simulink model "VehicleSilSimulation"  (R2026a)
settings: configuration reference "standardSILConfigurationParams" (kept outside this file)
StopFcn:
  | fid = fopen('C:\Users\Edison Altamirano\SITLV2\AnelloSummer\optimAeroPX4SIL\HILDiagnostics\logs\session_gtfix1\matlab_error_capture.txt','a'); fprintf(fid, '--- StopFcn fired at %s ---\n', datestr(now)); [m,i] = lasterr(); fprintf(fid, 'lasterr: %s (id: %s)\n', m, i); try; le = lasterror(); fprintf(fid, 'stack:\n'); for k=1:numel(le.stack); fprintf(fid, '  %s line %d\n', le.stack(k).name, le.stack(k).line); end; catch; end; fclose(fid);
values from neighbouring files (symbols this model uses):
  CONTROLLER_RUNTIME = 1    [initVehicleSIL.m]
  stepSize_s = 0.004    [initVehicleSIL.m]
  vehicleParams = evalin('base', 'vehicleParams')    [testVehicleSIL.m]
undefined symbols (not defined in the file or in its folder): actuatorDelay_s, controllerArmed, EngineCommandBus, gpsFreq, heartbeatFreq, opts, Payload, plantSampleTime_s, referenceLatitude_deg, referenceLongitude_deg, SampleTime, ServosCommandBus
libraries: uavmavlinklib x8, simulink x8, instrumentlib x6, flightGearInterfaceLibrary x6, aerolibfltsims x3, sharedtransform x3, px4MAVLinkBridgelib x2, aerolibanimutils x1, hdlsllib x1, dspnetwork x1, robotcorelib x1, uavutilslib x1
(part 2 of 3)

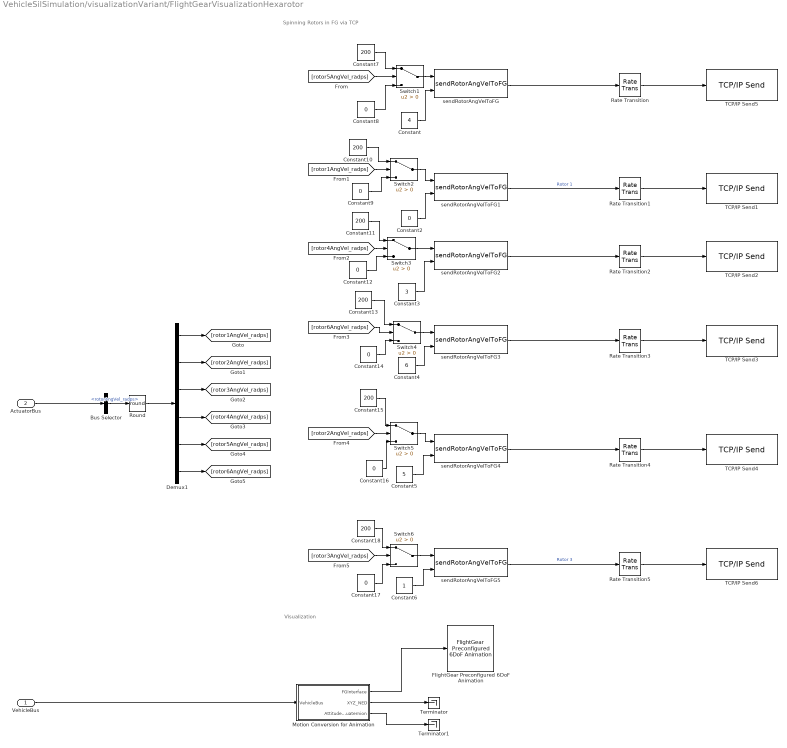
== system VehicleSilSimulation/visualizationVariant/FlightGearVisualizationHexarotor ==
  note: Spinning Rotors in FG via TCP
  note: Visualization
  VehicleBus : Inport
  ActuatorBus : Inport  Port=2  OutDataTypeStr=Bus:ActuatorBus
  Bus Selector : BusSelector  OutputSignals=PropulsionBus.rotorAngVel_radps
  Constant : Constant  Value=4
  Constant{7,10..11,13,15,18} (6 alike) : Constant  Value=200
  Constant{2,8..9,12,14,16..17} (7 alike) : Constant  Value=0
  Constant3 : Constant  Value=3
  Constant4 : Constant  Value=6
  Constant5 : Constant  Value=5
  Constant6 : Constant
  Demux1 : Demux  Outputs=6
  FlightGear Preconfigured 6DoF Animation : aerolibfltsims/FlightGear Preconfigured 6DoF Animation  xFlightGearVersion=v2019.1  DestinationIpAddress=127.0.0.1  DestinationPort=5502  SampleTime=-1  packetVersion=24
  Motion Conversion for Animation : Subsystem
      mask Display:
      | port_label('input',1,'ACBus')
      | port_label('output',1,'\lambda,L,h,\phi,\theta,\psi','texmode','on')
  Rate Transition{,1..5} (6 alike) : RateTransition  OutPortSampleTime=visualizationParams.flightGearFreq_Hz
  Round : Rounding  Operator=round
  Switch{1..6} (6 alike) : Switch  Criteria=u2 > Threshold  SaturateOnIntegerOverflow=off  InputSameDT=off
  TCP/IP Send{1..6} (6 alike) : instrumentlib/TCP//IP Send  Host=127.0.0.1  Port=5400  ByteOrder=big-endian  EnableBlockingMode=off  Timeout=10  TransferDelay=off  SimulateUsing=Interpreted execution
  Terminator : Terminator
  Terminator1 : Terminator
  sendRotorAngVelToFG{,1..5} (6 alike) : flightGearInterfaceLibrary/sendRotorAngVelToFG  SystemSampleTime=-1  VariantActivationTime=update diagram  EmptyChoice=off  PassThrough=off  PassThroughVariantControl=(default)  EmptyChoiceVariantControl=(default)  AllowFlexibleInterface=on  Latency=0  AutoFrameSizeCalculation=off
  wires:
  Motion Conversion for Animation/1(FGInterface) -> FlightGear Preconfigured 6DoF Animation/1
  VehicleBus/1 -> Motion Conversion for Animation/1(VehicleBus)
  Motion Conversion for Animation/2(XYZ_NED) -> Terminator/1
  Motion Conversion for Animation/3(AttitudeQuaternion) -> Terminator1/1
  ActuatorBus/1 -> Bus Selector/1
  Bus Selector/1 -> Round/1  "<rotorAngVel_radps>"
  Demux1/1 -> [rotor1AngVel_radps]
  Demux1/2 -> [rotor2AngVel_radps]
  Demux1/5 -> [rotor5AngVel_radps]
  Demux1/6 -> [rotor6AngVel_radps]
  Demux1/4 -> [rotor4AngVel_radps]
  Demux1/3 -> [rotor3AngVel_radps]
  Constant/1 -> sendRotorAngVelToFG/2
  Constant2/1 -> sendRotorAngVelToFG1/2
  Constant3/1 -> sendRotorAngVelToFG2/2
  Constant4/1 -> sendRotorAngVelToFG3/2
  Constant5/1 -> sendRotorAngVelToFG4/2
  Constant6/1 -> sendRotorAngVelToFG5/2
  Round/1 -> Demux1/1
  sendRotorAngVelToFG4/1 -> Rate Transition4/1
  sendRotorAngVelToFG3/1 -> Rate Transition3/1
  sendRotorAngVelToFG5/1 -> Rate Transition5/1  "Rotor 3"
  sendRotorAngVelToFG1/1 -> Rate Transition1/1  "Rotor 1"
  sendRotorAngVelToFG/1 -> Rate Transition/1
  sendRotorAngVelToFG2/1 -> Rate Transition2/1
  [rotor5AngVel_radps] -> Switch1/2
  Switch1/1 -> sendRotorAngVelToFG/1
  Constant7/1 -> Switch1/1
  Constant8/1 -> Switch1/3
  Switch2/1 -> sendRotorAngVelToFG1/1
  [rotor1AngVel_radps] -> Switch2/2
  Constant9/1 -> Switch2/3
  Constant10/1 -> Switch2/1
  Switch3/1 -> sendRotorAngVelToFG2/1
  [rotor4AngVel_radps] -> Switch3/2
  Constant11/1 -> Switch3/1
  Constant12/1 -> Switch3/3
  Switch4/1 -> sendRotorAngVelToFG3/1
  [rotor6AngVel_radps] -> Switch4/2
  Constant13/1 -> Switch4/1
  Constant14/1 -> Switch4/3
  Switch5/1 -> sendRotorAngVelToFG4/1
  [rotor2AngVel_radps] -> Switch5/2
  Constant15/1 -> Switch5/1
  Constant16/1 -> Switch5/3
  Switch6/1 -> sendRotorAngVelToFG5/1
  [rotor3AngVel_radps] -> Switch6/2
  Constant17/1 -> Switch6/3
  Constant18/1 -> Switch6/1
  Rate Transition/1 -> TCP/IP Send5/1
  Rate Transition1/1 -> TCP/IP Send1/1
  Rate Transition2/1 -> TCP/IP Send2/1
  Rate Transition3/1 -> TCP/IP Send3/1
  Rate Transition4/1 -> TCP/IP Send4/1
  Rate Transition5/1 -> TCP/IP Send6/1

== system VehicleSilSimulation/visualizationVariant/MatlabVisualization ==
  note: Visualization
  VehicleBus : Inport
  Motion Conversion for Animation : Subsystem
      mask Display:
      | port_label('input',1,'ACBus')
      | port_label('output',1,'\lambda,L,h,\phi,\theta,\psi','texmode','on')
  Terminator : Terminator
  UAV Animation : uavutilslib/UAV Animation  NumUAV=1  DynamicUAVConfig=off  UAVType=FixedWing  UAVSize=100  UAVColor=[1 0 0]  UAVTrajectoryAlpha=1  AlwaysShowAnimation=on  AxisLimits=[-Inf Inf;-Inf Inf;-Inf Inf]  TrajectoryBufferSize=100000  InertialZDirection=Down  RotationFormat=Quaternion  DrawMarkers=off  SampleTime=0.04
  wires:
  Motion Conversion for Animation/2(XYZ_NED) -> UAV Animation/1
  VehicleBus/1 -> Motion Conversion for Animation/1(VehicleBus)
  Motion Conversion for Animation/3(AttitudeQuaternion) -> UAV Animation/2
  Motion Conversion for Animation/1(FGInterface) -> Terminator/1

== system VehicleSilSimulation/visualizationVariant/passthrough ==
  VehicleBus : Inport
  Terminator : Terminator
  wires:
  VehicleBus/1 -> Terminator/1

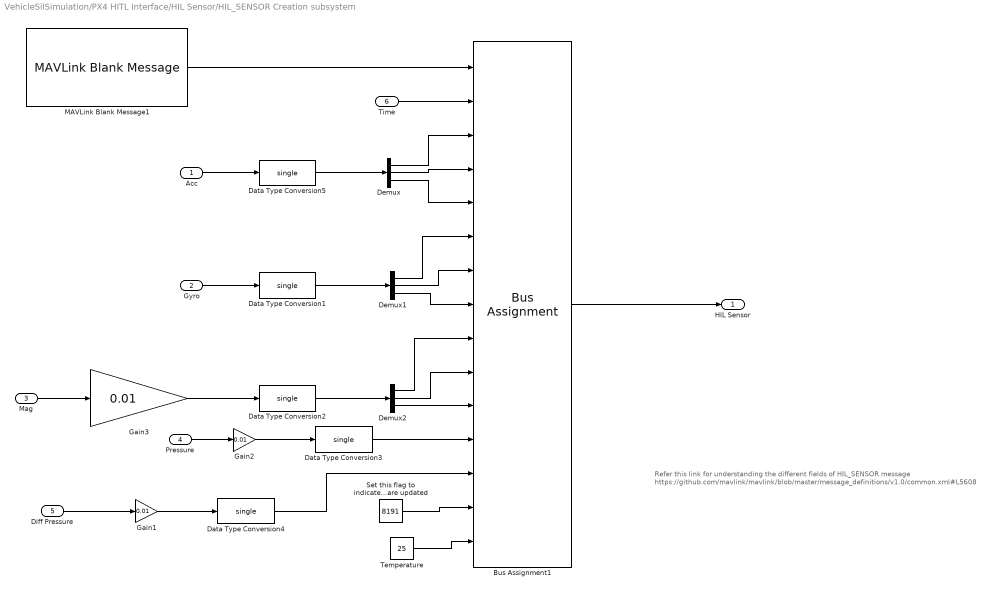
== system VehicleSilSimulation/PX4 HITL Interface/HIL Sensor/HIL_SENSOR Creation subsystem ==
  note: Refer this link for understanding the different fields of HIL_SENSOR message https://github.com/mavlink/mavlink/blob/master/message_definitions/v1.0/common.xml#L5608
  Acc : Inport
  Gyro : Inport  Port=2
  Mag : Inport  Port=3
  Pressure : Inport  Port=4
  Diff Pressure : Inport  Port=5
  Time : Inport  Port=6
  Bus Assignment1 : BusAssignment  AssignedSignals=Payload.time_usec,Payload.xacc,Payload.yacc,Payload.zacc,Payload.xgyro,Payload.ygyro,Payload.zgyro,Payload.xmag,Payload.ymag,Payload.zmag,Payload.abs_pressure,Payload.diff_pressure,Payload.fields_updated,Payload.temperature
  Data Type Conversion{1..5} (5 alike) : DataTypeConversion  OutDataTypeStr=single  SaturateOnIntegerOverflow=off  RndMeth=Floor
  Demux : Demux  Outputs=3
  Demux1 : Demux  Outputs=3
  Demux2 : Demux  Outputs=3
  Gain1 : Gain  Gain=0.01  OutDataTypeStr=single
  Gain2 : Gain  Gain=0.01  OutDataTypeStr=single
  Gain3 : Gain  Gain=0.01
  MAVLink Blank Message1 : uavmavlinklib/MAVLink Blank Message  dialectSource=Select from standard MAVLink dialects  dialect=common.xml  dialectCustom=common.xml  version=2  messageType=HIL_SENSOR  SystemID=2  ComponentID=51  SampleTime=-1
  Set this flag to indicate all flags are updated : Constant  Value=8191  OutDataTypeStr=Inherit: Inherit via back propagation  SampleTime=-1
  Temperature : Constant  Value=25  OutDataTypeStr=Inherit: Inherit via back propagation  SampleTime=-1
  HIL Sensor : Outport
  wires:
  Data Type Conversion2/1 -> Demux2/1
  Demux1/1 -> Bus Assignment1/6
  Mag/1 -> Gain3/1
  Demux1/3 -> Bus Assignment1/8
  Data Type Conversion1/1 -> Demux1/1
  Gyro/1 -> Data Type Conversion1/1
  Bus Assignment1/1 -> HIL Sensor/1
  Demux/3 -> Bus Assignment1/5
  Demux2/2 -> Bus Assignment1/10
  Demux2/3 -> Bus Assignment1/11
  Data Type Conversion5/1 -> Demux/1
  Demux/1 -> Bus Assignment1/3
  MAVLink Blank Message1/1 -> Bus Assignment1/1
  Demux2/1 -> Bus Assignment1/9
  Demux/2 -> Bus Assignment1/4
  Demux1/2 -> Bus Assignment1/7
  Acc/1 -> Data Type Conversion5/1
  Data Type Conversion3/1 -> Bus Assignment1/12
  Gain3/1 -> Data Type Conversion2/1
  Set this flag to indicate all flags are updated/1 -> Bus Assignment1/14
  Pressure/1 -> Gain2/1
  Time/1 -> Bus Assignment1/2
  Gain2/1 -> Data Type Conversion3/1
  Temperature/1 -> Bus Assignment1/15
  Diff Pressure/1 -> Gain1/1
  Gain1/1 -> Data Type Conversion4/1
  Data Type Conversion4/1 -> Bus Assignment1/13

== system VehicleSilSimulation/PX4 HITL Interface/HIL_GPS/GPS ==
  GPS Bytes : Inport
  Timestamp : Inport  Port=2
  Add : Sum  Inputs=+-
  Compare To Constant : simulink/Logic and Bit Operations/Compare To Constant  relop=>=  const=1e6*(1/gpsFreq)  OutDataTypeStr=uint8
  Compare To Constant1 : simulink/Logic and Bit Operations/Compare To Constant  relop=<  const=100000  OutDataTypeStr=boolean
  Constant : Constant  Value=0  OutDataTypeStr=uint8  SampleTime=SampleTime
  Data Store Read : DataStoreRead  DataStoreName=GPS  SampleTime=SampleTime  IndexOptions=Index vector (dialog)  Indices=1  OutputSizes=1
  GPS Time Update : Subsystem
  Logical Operator : Logic  Operator=OR  AllPortsSameDT=off  OutDataTypeStr=boolean
  Switch : Switch  Criteria=u2 > Threshold  SaturateOnIntegerOverflow=off  InputSameDT=off
  GPS Value : Outport
  Update GPS : Outport  Port=2
  wires:
  Timestamp/1 -> GPS Time Update/1(Timestamp), Compare To Constant1/1, Add/1
  Data Store Read/1 -> Add/2
  Add/1 -> Compare To Constant/1
  GPS Bytes/1 -> Switch/1
  Constant/1 -> Switch/3
  Switch/1 -> GPS Value/1
  Compare To Constant/1 -> Logical Operator/1
  Logical Operator/1 -> GPS Time Update/Enable, Update GPS/1, Switch/2
  Compare To Constant1/1 -> Logical Operator/2

== system VehicleSilSimulation/PX4 HITL Interface/HIL_GPS/GPS Serialization ==
  LLA : Inport
  Velocity : Inport  Port=2
  GndSpeed : Inport  Port=3
  Course : Inport  Port=4
  Time : Inport  Port=5
  Enable : EnablePort
  HIL_GPS Subsystem : Subsystem
  MAVLink Serializer3 : uavmavlinklib/MAVLink Serializer  dialectSource=Select from standard MAVLink dialects  dialect=common.xml  dialectCustom=common.xml  version=2  messageType=HIL_GPS
  Rate Transition : RateTransition  OutPortSampleTime=SampleTime
  Terminator : Terminator
  GPS Bytes : Outport
  wires:
  MAVLink Serializer3/1 -> GPS Bytes/1
  Velocity/1 -> HIL_GPS Subsystem/2(Velocity)
  Rate Transition/1 -> MAVLink Serializer3/1
  MAVLink Serializer3/2 -> Terminator/1
  HIL_GPS Subsystem/1(Out1) -> Rate Transition/1
  LLA/1 -> HIL_GPS Subsystem/1(LLA)
  Course/1 -> HIL_GPS Subsystem/4(Course)
  Time/1 -> HIL_GPS Subsystem/5(Time)
  GndSpeed/1 -> HIL_GPS Subsystem/3(GndSpeed)

== system VehicleSilSimulation/PX4 HITL Interface/Send Heartbeat/GPS ==
  Heartbeat Bytes : Inport
  Timestamp : Inport  Port=2
  Add : Sum  Inputs=+-
  Compare To Constant : simulink/Logic and Bit Operations/Compare To Constant  relop=>=  const=1e6*(1/heartbeatFreq)  OutDataTypeStr=uint8
  Compare To Constant1 : simulink/Logic and Bit Operations/Compare To Constant  relop=<  const=100000  OutDataTypeStr=boolean
  Constant : Constant  Value=0  OutDataTypeStr=uint8  SampleTime=SampleTime
  Data Store Read : DataStoreRead  DataStoreName=Heartbeat  SampleTime=SampleTime  IndexOptions=Index vector (dialog)  Indices=1  OutputSizes=1
  Heartbeat Time Update : Subsystem
  Logical Operator : Logic  Operator=OR  AllPortsSameDT=off  OutDataTypeStr=boolean
  Switch : Switch  Criteria=u2 > Threshold  SaturateOnIntegerOverflow=off  InputSameDT=off
  Update Heartbeat : Outport
  Heartbeat Value : Outport  Port=2
  wires:
  Timestamp/1 -> Heartbeat Time Update/1(Timestamp), Compare To Constant1/1, Add/1
  Data Store Read/1 -> Add/2
  Add/1 -> Compare To Constant/1
  Heartbeat Bytes/1 -> Switch/1
  Constant/1 -> Switch/3
  Switch/1 -> Heartbeat Value/1
  Compare To Constant1/1 -> Logical Operator/2
  Compare To Constant/1 -> Logical Operator/1
  Logical Operator/1 -> Switch/2, Update Heartbeat/1, Heartbeat Time Update/Enable

== system VehicleSilSimulation/PX4 HITL Interface/Send Heartbeat/Heartbeat_Serialization ==
  Enable : EnablePort
  Bus Assignment : BusAssignment  AssignedSignals=Payload.autopilot,Payload.type
  Constant : Constant  SampleTime=-1
  Constant1 : Constant  Value=12  SampleTime=-1
  Data Type Conversion : DataTypeConversion  OutDataTypeStr=uint8  SaturateOnIntegerOverflow=off  RndMeth=Floor
  Data Type Conversion1 : DataTypeConversion  OutDataTypeStr=uint8  SaturateOnIntegerOverflow=off  RndMeth=Floor
  MAVLink Blank Message : uavmavlinklib/MAVLink Blank Message  dialectSource=Select from standard MAVLink dialects  dialect=common.xml  dialectCustom=common.xml  version=2  messageType=HEARTBEAT  SystemID=2  ComponentID=51  SampleTime=SampleTime
  MAVLink Serializer : uavmavlinklib/MAVLink Serializer  dialectSource=Select from standard MAVLink dialects  dialect=common.xml  dialectCustom=common.xml  version=2  messageType=HEARTBEAT
  Terminator4 : Terminator
  Heartbeat : Outport
  wires:
  Data Type Conversion1/1 -> Bus Assignment/3
  Constant/1 -> Data Type Conversion/1
  Constant1/1 -> Data Type Conversion1/1
  Bus Assignment/1 -> MAVLink Serializer/1
  MAVLink Serializer/2 -> Terminator4/1
  Data Type Conversion/1 -> Bus Assignment/2
  MAVLink Blank Message/1 -> Bus Assignment/1
  MAVLink Serializer/1 -> Heartbeat/1

== system VehicleSilSimulation/vehicleSimulation/plant/Add Custom Aircraft Plant HERE ==
  ActuatorCommandBus : Inport
  InitialConditionBus : Inport  Port=2
  EnvironmentBus : Inport  Port=3
  VehicleBus : Outport
  ActuatorBus : Outport  Port=2  OutDataTypeStr=Bus: ActuatorBus

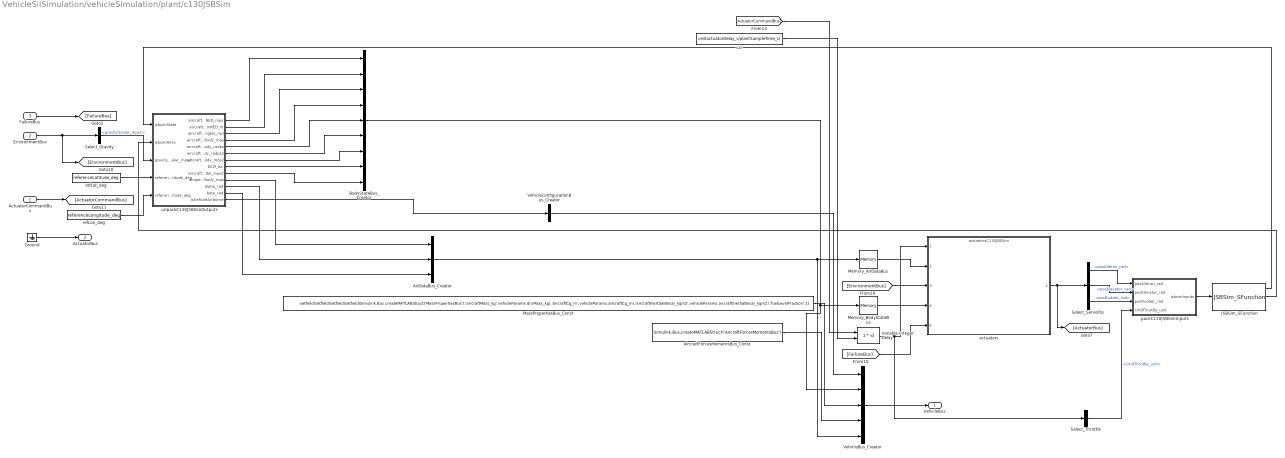
== system VehicleSilSimulation/vehicleSimulation/plant/c130JSBSim ==
  ActuatorCommandBus : Inport  OutDataTypeStr=Bus: ActuatorCommandBus
  EnvironmentBus : Inport  Port=2  OutDataTypeStr=Bus: EnvironmentBus
  FailureBus : Inport  Port=3  OutDataTypeStr=Bus: FailureBus
  AirDataBus_Creator : BusCreator  Inputs=3  OutDataTypeStr=Bus: AirDataBus
  AircraftForcesMomentsBus_Const : Constant  Value=Simulink.Bus.createMATLABStruct('AircraftForcesMomentsBus')  OutDataTypeStr=Bus: AircraftForcesMomentsBus
  BodyStateBus_Creator : BusCreator  Inputs=9  OutDataTypeStr=Bus: BodyStateBus
  Ground : Ground
  JSBSim_SFunction : S-Function  FunctionName=JSBSim_SFunction  Parameters='C130', stepSize_s, 0, '', 'c130JSBSimInit', 'C:/Users/Edison Altamirano/SITLV2/AnelloSummer/optimAeroPX4SIL/c130JSBSim_io.xml'  SFunctionDeploymentMode=off  EnableBusSupport=off
  MassPropertiesBus_Const : Constant  Value=setfield(setfield(setfield(setfield(Simulink.Bus.createMATLABStruct('MassPropertiesBus'),'aircraftMass_kg',vehicleParams.dryMass_kg),'aircraftCg_m',vehicleParams.aircraftCg_m),'aircraftInertiaInBody_kgm2',vehicleParams.aircraftInertialBody_kgm2),'fuelLevelFraction',1)  OutDataTypeStr=Bus: MassPropertiesBus
  Memory_AirDataBus : Memory
  Memory_BodyStateBus : Memory
  Select_Gravity : BusSelector  OutputSignals=EarthEnvironment.gravityScalar_mps2
  Select_ServoPos : BusSelector  OutputSignals=ServosBus.ServosFixedwingPlaneBus.posAileron_rad,ServosBus.ServosFixedwingPlaneBus.posElevator_rad,ServosBus.ServosFixedwingPlaneBus.posRudder_rad
  Select_Throttle : BusSelector  OutputSignals=EngineCommandBus.cmdThrottle_unit
  Variable Integer Delay : Delay  DelayLengthSource=Input port
      settings: InputPortMap=u0,p1
  VehicleBus_Creator : BusCreator  Inputs=5  OutDataTypeStr=Bus: VehicleBus
  VehicleConfigurationBus_Creator : BusCreator  Inputs=1  OutDataTypeStr=Bus: VehicleConfigurationBus
  actuators : ModelReference  ModelNameDialog=actuatorsC130JSBSim.slx  SimulationMode=Normal  ModelReferenceVersion=5.3
  packC130JSBSimInputs : MATLAB Function  TreatAsAtomicUnit=on
  refLat_deg : Constant  Value=referenceLatitude_deg
  refLon_deg : Constant  Value=referenceLongitude_deg
  unpackC130JSBSimOutputs : MATLAB Function  TreatAsAtomicUnit=on
  var : Constant  Value=ceil(actuatorDelay_s/plantSampleTime_s)
  VehicleBus : Outport  OutDataTypeStr=Bus: VehicleBus
  ActuatorBus : Outport  Port=2  OutDataTypeStr=Bus: ActuatorBus
  wires:
  Select_Throttle/1 -> packC130JSBSimInputs/4(cmdThrottle_unit)  "<cmdThrottle_unit>"
  JSBSim_SFunction/1 -> unpackC130JSBSimOutputs/1(jsbsimState)
  Select_ServoPos/3 -> packC130JSBSimInputs/3(posRudder_rad)  "<posRudder_rad>"
  Select_ServoPos/1 -> packC130JSBSimInputs/1(posAileron_rad)  "<posAileron_rad>"
  actuators/1 -> [ActuatorBus], Select_ServoPos/1
  VehicleBus_Creator/1 -> VehicleBus/1
  Select_ServoPos/2 -> packC130JSBSimInputs/2(posElevator_rad)  "<posElevator_rad>"
  Memory_AirDataBus/1 -> actuators/2
  AircraftForcesMomentsBus_Const/1 -> VehicleBus_Creator/4
  AirDataBus_Creator/1 -> Memory_AirDataBus/1, VehicleBus_Creator/5
  BodyStateBus_Creator/1 -> Memory_BodyStateBus/1, VehicleBus_Creator/2
  JSBSim_SFunction/2 -> unpackC130JSBSimOutputs/2(jsbsimAero)
  var/1 -> Variable Integer Delay/2
  packC130JSBSimInputs/1(jsbsimInputs) -> JSBSim_SFunction/1
  [ActuatorCommandBus] -> Variable Integer Delay/1
  Memory_BodyStateBus/1 -> actuators/4
  unpackC130JSBSimOutputs/13(isVehicleAirborne) -> VehicleConfigurationBus_Creator/1
  unpackC130JSBSimOutputs/12(beta_rad) -> AirDataBus_Creator/3
  unpackC130JSBSimOutputs/11(alpha_rad) -> AirDataBus_Creator/2
  unpackC130JSBSimOutputs/10(airspeedInBody_mps) -> AirDataBus_Creator/1
  unpackC130JSBSimOutputs/9(aircraftAccelbe_mps2) -> BodyStateBus_Creator/9
  unpackC130JSBSimOutputs/8(DCM_be) -> BodyStateBus_Creator/8
  VehicleConfigurationBus_Creator/1 -> VehicleBus_Creator/1
  unpackC130JSBSimOutputs/7(aircraftAccelInBody_mps2) -> BodyStateBus_Creator/7
  unpackC130JSBSimOutputs/6(aircraftAngAccelInBody_radps2) -> BodyStateBus_Creator/6
  unpackC130JSBSimOutputs/5(aircraftAngVelInBody_radps) -> BodyStateBus_Creator/5
  unpackC130JSBSimOutputs/4(aircraftVelInBody_mps) -> BodyStateBus_Creator/4
  unpackC130JSBSimOutputs/2(aircraftPosInNED_m) -> BodyStateBus_Creator/2
  unpackC130JSBSimOutputs/3(aircraftEulerAngles_rad) -> BodyStateBus_Creator/3
  refLon_deg/1 -> unpackC130JSBSimOutputs/5(referenceLongitude_deg)
  refLat_deg/1 -> unpackC130JSBSimOutputs/4(referenceLatitude_deg)
  unpackC130JSBSimOutputs/1(aircraftVelInNED_mps) -> BodyStateBus_Creator/1
  Ground/1 -> ActuatorBus/1
  ActuatorCommandBus/1 -> [ActuatorCommandBus]
  MassPropertiesBus_Const/1 -> VehicleBus_Creator/3
  Select_Gravity/1 -> unpackC130JSBSimOutputs/3(gravityScalar_mps2)  "<gravityScalar_mps2>"
  FailureBus/1 -> [FailureBus]
  [EnvironmentBus] -> actuators/3
  Variable Integer Delay/1 -> actuators/1, Select_Throttle/1
  EnvironmentBus/1 -> [EnvironmentBus], Select_Gravity/1
  [FailureBus] -> actuators/5

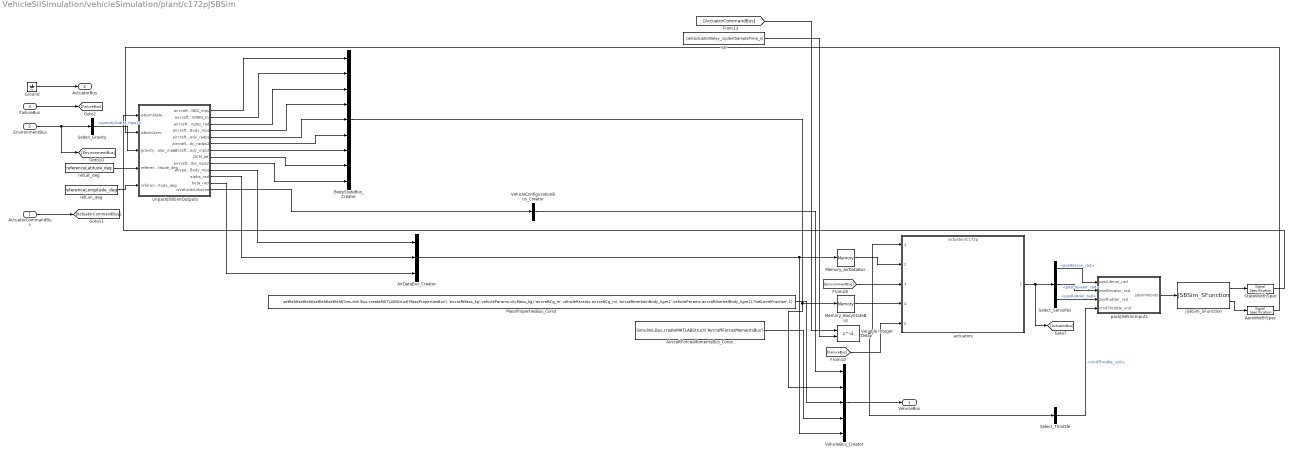
== system VehicleSilSimulation/vehicleSimulation/plant/c172pJSBSim ==
  ActuatorCommandBus : Inport  OutDataTypeStr=Bus: ActuatorCommandBus
  EnvironmentBus : Inport  Port=2  OutDataTypeStr=Bus: EnvironmentBus
  FailureBus : Inport  Port=3  OutDataTypeStr=Bus: FailureBus
  AeroWidthSpec : SignalSpecification  Dimensions=5
  AirDataBus_Creator : BusCreator  Inputs=3  OutDataTypeStr=Bus: AirDataBus
  AircraftForcesMomentsBus_Const : Constant  Value=Simulink.Bus.createMATLABStruct('AircraftForcesMomentsBus')  OutDataTypeStr=Bus: AircraftForcesMomentsBus
  BodyStateBus_Creator : BusCreator  Inputs=9  OutDataTypeStr=Bus: BodyStateBus
  Ground : Ground
  JSBSim_SFunction : S-Function  FunctionName=JSBSim_SFunction  Parameters='c172p', stepSize_s, 0, '', 'c172pJSBSimInit', 'C:/SITL/AnelloSummer/optimAeroPX4SIL/c172pJSBSim_io.xml'  SFunctionDeploymentMode=off  EnableBusSupport=off
  MassPropertiesBus_Const : Constant  Value=setfield(setfield(setfield(setfield(Simulink.Bus.createMATLABStruct('MassPropertiesBus'),'aircraftMass_kg',vehicleParams.dryMass_kg),'aircraftCg_m',vehicleParams.aircraftCg_m),'aircraftInertiaInBody_kgm2',vehicleParams.aircraftInertialBody_kgm2),'fuelLevelFraction',1)  OutDataTypeStr=Bus: MassPropertiesBus
  Memory_AirDataBus : Memory
  Memory_BodyStateBus : Memory
  Select_Gravity : BusSelector  OutputSignals=EarthEnvironment.gravityScalar_mps2
  Select_ServoPos : BusSelector  OutputSignals=ServosBus.ServosFixedwingPlaneBus.posAileron_rad,ServosBus.ServosFixedwingPlaneBus.posElevator_rad,ServosBus.ServosFixedwingPlaneBus.posRudder_rad
  Select_Throttle : BusSelector  OutputSignals=EngineCommandBus.cmdThrottle_unit
  StateWidthSpec : SignalSpecification  Dimensions=19
  Variable Integer Delay : Delay  DelayLengthSource=Input port
      settings: InputPortMap=u0,p1
  VehicleBus_Creator : BusCreator  Inputs=5  OutDataTypeStr=Bus: VehicleBus
  VehicleConfigurationBus_Creator : BusCreator  Inputs=1  OutDataTypeStr=Bus: VehicleConfigurationBus
  actuators : ModelReference  ModelNameDialog=actuatorsC172p.slx  SimulationMode=Normal  ModelReferenceVersion=5.3
  packJSBSimInputs : MATLAB Function  TreatAsAtomicUnit=on
  refLat_deg : Constant  Value=referenceLatitude_deg
  refLon_deg : Constant  Value=referenceLongitude_deg
  unpackJSBSimOutputs : MATLAB Function  TreatAsAtomicUnit=on
  var : Constant  Value=ceil(actuatorDelay_s/plantSampleTime_s)
  VehicleBus : Outport  OutDataTypeStr=Bus: VehicleBus
  ActuatorBus : Outport  Port=2  OutDataTypeStr=Bus: ActuatorBus
  wires:
  StateWidthSpec/1 -> unpackJSBSimOutputs/1(jsbsimState)
  JSBSim_SFunction/1 -> StateWidthSpec/1
  packJSBSimInputs/1(jsbsimInputs) -> JSBSim_SFunction/1
  Select_Throttle/1 -> packJSBSimInputs/4(cmdThrottle_unit)  "<cmdThrottle_unit>"
  AeroWidthSpec/1 -> unpackJSBSimOutputs/2(jsbsimAero)
  Select_ServoPos/3 -> packJSBSimInputs/3(posRudder_rad)  "<posRudder_rad>"
  Select_ServoPos/2 -> packJSBSimInputs/2(posElevator_rad)  "<posElevator_rad>"
  Select_ServoPos/1 -> packJSBSimInputs/1(posAileron_rad)  "<posAileron_rad>"
  actuators/1 -> [ActuatorBus], Select_ServoPos/1
  VehicleBus_Creator/1 -> VehicleBus/1
  Variable Integer Delay/1 -> Select_Throttle/1, actuators/1
  Memory_BodyStateBus/1 -> actuators/4
  AircraftForcesMomentsBus_Const/1 -> VehicleBus_Creator/4
  MassPropertiesBus_Const/1 -> VehicleBus_Creator/3
  Memory_AirDataBus/1 -> actuators/2
  AirDataBus_Creator/1 -> Memory_AirDataBus/1, VehicleBus_Creator/5
  VehicleConfigurationBus_Creator/1 -> VehicleBus_Creator/1
  var/1 -> Variable Integer Delay/2
  unpackJSBSimOutputs/13(isVehicleAirborne) -> VehicleConfigurationBus_Creator/1
  unpackJSBSimOutputs/12(beta_rad) -> AirDataBus_Creator/3
  unpackJSBSimOutputs/11(alpha_rad) -> AirDataBus_Creator/2
  [FailureBus] -> actuators/5
  unpackJSBSimOutputs/10(airspeedInBody_mps) -> AirDataBus_Creator/1
  unpackJSBSimOutputs/9(aircraftAccelbe_mps2) -> BodyStateBus_Creator/9
  unpackJSBSimOutputs/8(DCM_be) -> BodyStateBus_Creator/8
  unpackJSBSimOutputs/6(aircraftAngAccelInBody_radps2) -> BodyStateBus_Creator/6
  unpackJSBSimOutputs/5(aircraftAngVelInBody_radps) -> BodyStateBus_Creator/5
  unpackJSBSimOutputs/4(aircraftVelInBody_mps) -> BodyStateBus_Creator/4
  unpackJSBSimOutputs/3(aircraftEulerAngles_rad) -> BodyStateBus_Creator/3
  [ActuatorCommandBus] -> Variable Integer Delay/1
  unpackJSBSimOutputs/2(aircraftPosInNED_m) -> BodyStateBus_Creator/2
  [EnvironmentBus] -> actuators/3
  unpackJSBSimOutputs/1(aircraftVelInNED_mps) -> BodyStateBus_Creator/1
  refLat_deg/1 -> unpackJSBSimOutputs/4(referenceLatitude_deg)
  refLon_deg/1 -> unpackJSBSimOutputs/5(referenceLongitude_deg)
  EnvironmentBus/1 -> [EnvironmentBus], Select_Gravity/1
  ActuatorCommandBus/1 -> [ActuatorCommandBus]
  BodyStateBus_Creator/1 -> Memory_BodyStateBus/1, VehicleBus_Creator/2
  Select_Gravity/1 -> unpackJSBSimOutputs/3(gravityScalar_mps2)  "<gravityScalar_mps2>"
  FailureBus/1 -> [FailureBus]
  unpackJSBSimOutputs/7(aircraftAccelInBody_mps2) -> BodyStateBus_Creator/7
  Ground/1 -> ActuatorBus/1
  JSBSim_SFunction/2 -> AeroWidthSpec/1

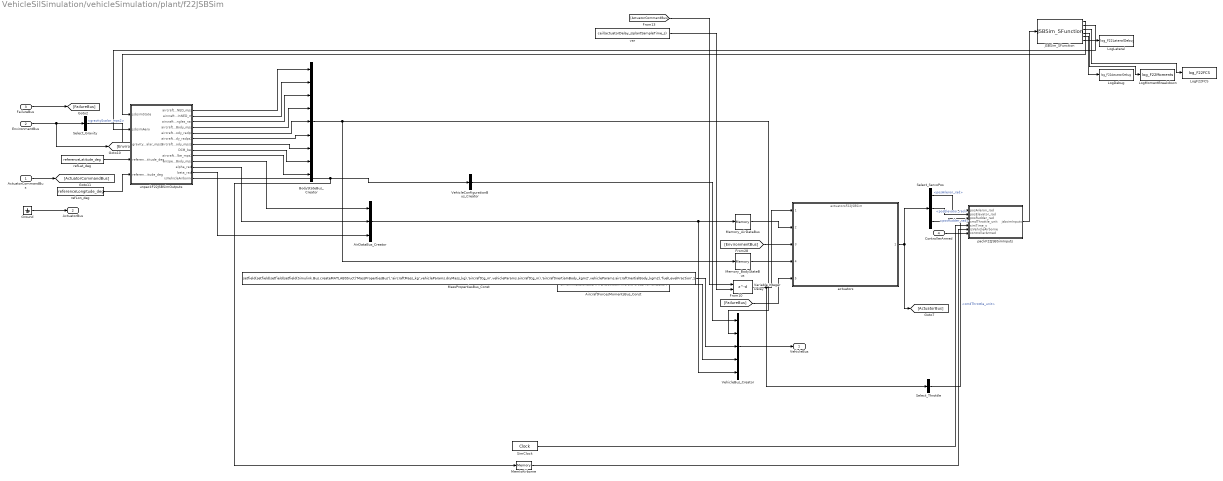
== system VehicleSilSimulation/vehicleSimulation/plant/f22JSBSim ==
  ActuatorCommandBus : Inport  OutDataTypeStr=Bus: ActuatorCommandBus
  EnvironmentBus : Inport  Port=2  OutDataTypeStr=Bus: EnvironmentBus
  FailureBus : Inport  Port=3  OutDataTypeStr=Bus: FailureBus
  ControllerArmed : Inport  Port=4
  AirDataBus_Creator : BusCreator  Inputs=3  OutDataTypeStr=Bus: AirDataBus
  AircraftForcesMomentsBus_Const : Constant  Value=Simulink.Bus.createMATLABStruct('AircraftForcesMomentsBus')  OutDataTypeStr=Bus: AircraftForcesMomentsBus
  BodyStateBus_Creator : BusCreator  Inputs=9  OutDataTypeStr=Bus: BodyStateBus
  Ground : Ground
  JSBSim_SFunction : S-Function  FunctionName=JSBSim_SFunction  Parameters='f22', stepSize_s, 0, '', 'f22JSBSimInit', 'C:/Users/Edison Altamirano/SITLV2/AnelloSummer/optimAeroPX4SIL/f22JSBSim_io.xml'  SFunctionDeploymentMode=off  EnableBusSupport=off
  LogDebug : ToWorkspace  VariableName=log_F22ActuatorDebug  SaveFormat=Structure With Time
  LogF22FCS : ToWorkspace  VariableName=log_F22FCS  SaveFormat=Structure With Time  SampleTime=-1
  LogLateral : ToWorkspace  VariableName=log_F22LateralDebug  SaveFormat=Structure With Time
  LogMomentBreakdown : ToWorkspace  VariableName=log_F22Moments  SaveFormat=Structure With Time
  MassPropertiesBus_Const : Constant  Value=setfield(setfield(setfield(setfield(Simulink.Bus.createMATLABStruct('MassPropertiesBus'),'aircraftMass_kg',vehicleParams.dryMass_kg),'aircraftCg_m',vehicleParams.aircraftCg_m),'aircraftInertiaInBody_kgm2',vehicleParams.aircraftInertialBody_kgm2),'fuelLevelFraction',1)  OutDataTypeStr=Bus: MassPropertiesBus
  MemIsAirborne : Memory
  Memory_AirDataBus : Memory
  Memory_BodyStateBus : Memory
  Select_Gravity : BusSelector  OutputSignals=EarthEnvironment.gravityScalar_mps2
  Select_ServoPos : BusSelector  OutputSignals=ServosBus.ServosFixedwingPlaneBus.posAileron_rad,ServosBus.ServosFixedwingPlaneBus.posElevator_rad,ServosBus.ServosFixedwingPlaneBus.posRudder_rad
  Select_Throttle : BusSelector  OutputSignals=EngineCommandBus.cmdThrottle_unit
  SimClock : DigitalClock  SampleTime=stepSize_s
  Variable Integer Delay : Delay  DelayLengthSource=Input port
      settings: InputPortMap=u0,p1
  VehicleBus_Creator : BusCreator  Inputs=5  OutDataTypeStr=Bus: VehicleBus
  VehicleConfigurationBus_Creator : BusCreator  Inputs=1  OutDataTypeStr=Bus: VehicleConfigurationBus
  actuators : ModelReference  ModelNameDialog=actuatorsF22JSBSim  SimulationMode=Normal  ModelReferenceVersion=5.3
  packF22JSBSimInputs : MATLAB Function  TreatAsAtomicUnit=on  SystemSampleTime=stepSize_s
  refLat_deg : Constant  Value=referenceLatitude_deg
  refLon_deg : Constant  Value=referenceLongitude_deg
  unpackF22JSBSimOutputs : MATLAB Function  TreatAsAtomicUnit=on
  var : Constant  Value=ceil(actuatorDelay_s/plantSampleTime_s)
  VehicleBus : Outport  OutDataTypeStr=Bus: VehicleBus
  ActuatorBus : Outport  Port=2  OutDataTypeStr=Bus: ActuatorBus
  wires:
  JSBSim_SFunction/4 -> LogMomentBreakdown/1
  JSBSim_SFunction/3 -> LogF22FCS/1
  SimClock/1 -> packF22JSBSimInputs/5(simTime_s)
  MemIsAirborne/1 -> packF22JSBSimInputs/6(isVehicleAirborne)
  Select_Throttle/1 -> packF22JSBSimInputs/4(cmdThrottle_unit)  "<cmdThrottle_unit>"
  JSBSim_SFunction/2 -> unpackF22JSBSimOutputs/2(jsbsimAero)
  JSBSim_SFunction/1 -> unpackF22JSBSimOutputs/1(jsbsimState)
  packF22JSBSimInputs/1(jsbsimInputs) -> JSBSim_SFunction/1
  Select_ServoPos/3 -> packF22JSBSimInputs/3(posRudder_rad)  "<posRudder_rad>"
  Select_ServoPos/1 -> packF22JSBSimInputs/1(posAileron_rad)  "<posAileron_rad>"
  actuators/1 -> [ActuatorBus], Select_ServoPos/1
  Variable Integer Delay/1 -> Select_Throttle/1, actuators/1
  AircraftForcesMomentsBus_Const/1 -> VehicleBus_Creator/4
  MassPropertiesBus_Const/1 -> VehicleBus_Creator/3
  Memory_AirDataBus/1 -> actuators/2
  [EnvironmentBus] -> actuators/3
  VehicleConfigurationBus_Creator/1 -> VehicleBus_Creator/1
  BodyStateBus_Creator/1 -> Memory_BodyStateBus/1, VehicleBus_Creator/2
  [ActuatorCommandBus] -> Variable Integer Delay/1
  AirDataBus_Creator/1 -> Memory_AirDataBus/1, VehicleBus_Creator/5
  unpackF22JSBSimOutputs/13(isVehicleAirborne) -> MemIsAirborne/1, VehicleConfigurationBus_Creator/1
  unpackF22JSBSimOutputs/12(beta_rad) -> AirDataBus_Creator/3
  unpackF22JSBSimOutputs/11(alpha_rad) -> AirDataBus_Creator/2
  unpackF22JSBSimOutputs/10(airspeedInBody_mps) -> AirDataBus_Creator/1
  unpackF22JSBSimOutputs/9(aircraftAccelbe_mps2) -> BodyStateBus_Creator/9
  unpackF22JSBSimOutputs/8(DCM_be) -> BodyStateBus_Creator/8
  Memory_BodyStateBus/1 -> actuators/4
  unpackF22JSBSimOutputs/7(aircraftAccelInBody_mps2) -> BodyStateBus_Creator/7
  unpackF22JSBSimOutputs/6(aircraftAngAccelInBody_radps2) -> BodyStateBus_Creator/6
  unpackF22JSBSimOutputs/5(aircraftAngVelInBody_radps) -> BodyStateBus_Creator/5
  unpackF22JSBSimOutputs/4(aircraftVelInBody_mps) -> BodyStateBus_Creator/4
  unpackF22JSBSimOutputs/3(aircraftEulerAngles_rad) -> BodyStateBus_Creator/3
  unpackF22JSBSimOutputs/2(aircraftPosInNED_m) -> BodyStateBus_Creator/2
  unpackF22JSBSimOutputs/1(aircraftVelInNED_mps) -> BodyStateBus_Creator/1
  Select_Gravity/1 -> unpackF22JSBSimOutputs/3(gravityScalar_mps2)  "<gravityScalar_mps2>"
  Ground/1 -> ActuatorBus/1
  EnvironmentBus/1 -> [EnvironmentBus], Select_Gravity/1
  Select_ServoPos/2 -> packF22JSBSimInputs/2(posElevator_rad)  "<posElevator_rad>"
  refLon_deg/1 -> unpackF22JSBSimOutputs/5(referenceLongitude_deg)
  FailureBus/1 -> [FailureBus]
  VehicleBus_Creator/1 -> VehicleBus/1
  ActuatorCommandBus/1 -> [ActuatorCommandBus]
  refLat_deg/1 -> unpackF22JSBSimOutputs/4(referenceLatitude_deg)
  var/1 -> Variable Integer Delay/2
  [FailureBus] -> actuators/5
  JSBSim_SFunction/5 -> LogDebug/1
  ControllerArmed/1 -> packF22JSBSimInputs/7(controllerArmed)
  JSBSim_SFunction/6 -> LogLateral/1

== system VehicleSilSimulation/visualizationVariant/FlightGearVisualizationF16/Motion Conversion for Animation ==
  VehicleBus : Inport  OutDataTypeStr=Bus: VehicleBus
  Bus Selector : BusSelector  OutputSignals=BodyStatesBus.aircraftEulerAngles_rad
  Bus Selector1 : BusSelector  OutputSignals=BodyStatesBus.aircraftPosInNED_m
  Constant : Constant  Value=0
  Flat Earth to LLA : FlatEarth2LLA  R=6378137  LL0=[referenceLatitude_deg, referenceLongitude_deg]
  Mux : Mux  Inputs=2
  Mux1 : Mux  Inputs=2
  Rotation Angles to Quaternions : sharedtransform/Rotation Angles to Quaternions  rotationOrder=ZYX  aMode=aMode
  Selector : Selector  IndexMode=Zero-based  InputPortWidth=2  IndexOptions=Index vector (dialog)  Indices=[1 0]  OutputSizes=1
  FGInterface : Outport  VectorParamsAs1DForOutWhenUnconnected=off
  XYZ_NED : Outport  Port=2  VectorParamsAs1DForOutWhenUnconnected=off
  AttitudeQuaternion : Outport  Port=3  VectorParamsAs1DForOutWhenUnconnected=off
  wires:
  Mux1/1 -> FGInterface/1
  Constant/1 -> Flat Earth to LLA/2
  Bus Selector/1 -> Rotation Angles to Quaternions/1, Mux1/2  "<aircraftEulerAngles_rad>"
  Flat Earth to LLA/2 -> Mux/2
  Flat Earth to LLA/1 -> Selector/1
  Bus Selector1/1 -> Flat Earth to LLA/1  "<aircraftPosInNED_m>"
  VehicleBus/1 -> Bus Selector/1, Bus Selector1/1
  Selector/1 -> Mux/1
  Mux/1 -> XYZ_NED/1, Mux1/1
  Rotation Angles to Quaternions/1 -> AttitudeQuaternion/1

== system VehicleSilSimulation/visualizationVariant/FlightGearVisualizationFixedWing/Motion Conversion for Animation ==
  VehicleBus : Inport  OutDataTypeStr=Bus: VehicleBus
  Bus Selector : BusSelector  OutputSignals=BodyStatesBus.aircraftEulerAngles_rad
  Bus Selector1 : BusSelector  OutputSignals=BodyStatesBus.aircraftPosInNED_m
  Constant : Constant  Value=0
  Flat Earth to LLA : FlatEarth2LLA  R=6378137  LL0=[referenceLatitude_deg, referenceLongitude_deg]
  Mux : Mux  Inputs=2
  Mux1 : Mux  Inputs=2
  Rotation Angles to Quaternions : sharedtransform/Rotation Angles to Quaternions  rotationOrder=ZYX  aMode=aMode
  Selector : Selector  IndexMode=Zero-based  InputPortWidth=2  IndexOptions=Index vector (dialog)  Indices=[1 0]  OutputSizes=1
  FGInterface : Outport  VectorParamsAs1DForOutWhenUnconnected=off
  XYZ_NED : Outport  Port=2  VectorParamsAs1DForOutWhenUnconnected=off
  AttitudeQuaternion : Outport  Port=3  VectorParamsAs1DForOutWhenUnconnected=off
  wires:
  Rotation Angles to Quaternions/1 -> AttitudeQuaternion/1
  Mux/1 -> Mux1/1, XYZ_NED/1
  Selector/1 -> Mux/1
  VehicleBus/1 -> Bus Selector1/1, Bus Selector/1
  Bus Selector1/1 -> Flat Earth to LLA/1  "<aircraftPosInNED_m>"
  Flat Earth to LLA/1 -> Selector/1
  Flat Earth to LLA/2 -> Mux/2
  Bus Selector/1 -> Mux1/2, Rotation Angles to Quaternions/1  "<aircraftEulerAngles_rad>"
  Constant/1 -> Flat Earth to LLA/2
  Mux1/1 -> FGInterface/1

== system VehicleSilSimulation/visualizationVariant/FlightGearVisualizationHexarotor/Motion Conversion for Animation ==
  VehicleBus : Inport  OutDataTypeStr=Bus: VehicleBus
  Bus Selector : BusSelector  OutputSignals=BodyStatesBus.aircraftEulerAngles_rad
  Bus Selector1 : BusSelector  OutputSignals=BodyStatesBus.aircraftPosInNED_m
  Constant : Constant  Value=0
  Flat Earth to LLA : FlatEarth2LLA  R=6378137  LL0=[referenceLatitude_deg, referenceLongitude_deg]
  Mux : Mux  Inputs=2
  Mux1 : Mux  Inputs=2
  Rotation Angles to Quaternions : sharedtransform/Rotation Angles to Quaternions  rotationOrder=ZYX  aMode=aMode
  Selector : Selector  IndexMode=Zero-based  InputPortWidth=2  IndexOptions=Index vector (dialog)  Indices=[1 0]  OutputSizes=1
  FGInterface : Outport  VectorParamsAs1DForOutWhenUnconnected=off
  XYZ_NED : Outport  Port=2  VectorParamsAs1DForOutWhenUnconnected=off
  AttitudeQuaternion : Outport  Port=3  VectorParamsAs1DForOutWhenUnconnected=off
  wires:
  Mux1/1 -> FGInterface/1
  Constant/1 -> Flat Earth to LLA/2
  Bus Selector/1 -> Rotation Angles to Quaternions/1, Mux1/2  "<aircraftEulerAngles_rad>"
  Flat Earth to LLA/2 -> Mux/2
  Flat Earth to LLA/1 -> Selector/1
  Bus Selector1/1 -> Flat Earth to LLA/1  "<aircraftPosInNED_m>"
  VehicleBus/1 -> Bus Selector/1, Bus Selector1/1
  Selector/1 -> Mux/1
  Mux/1 -> XYZ_NED/1, Mux1/1
  Rotation Angles to Quaternions/1 -> AttitudeQuaternion/1

== system VehicleSilSimulation/visualizationVariant/MatlabVisualization/Motion Conversion for Animation ==
  VehicleBus : Inport  OutDataTypeStr=Bus: VehicleBus
  Bus Selector : BusSelector  OutputSignals=signal2.aircraftEulerAngles_rad
  Bus Selector1 : BusSelector  OutputSignals=signal2.aircraftPosInNED_m
  Constant : Constant  Value=0
  Coordinate Transformation Conversion : robotcorelib/Coordinate Transformation Conversion  InputRepresentation=Euler Angles  InputEulerSequence=XYZ  ShowTrVecInputPort=on  OutputRepresentation=Quaternion  OutputEulerSequence=ZYX  ShowTrVecOutputPort=on  SimulateUsing=Code generation
  Flat Earth to LLA : FlatEarth2LLA  R=6378137  LL0=[referenceLatitude_deg, referenceLongitude_deg]
  Gain : Gain  Gain=-1
  Mux : Mux  Inputs=2
  Mux1 : Mux  Inputs=2
  Selector : Selector  IndexMode=Zero-based  InputPortWidth=2  IndexOptions=Index vector (dialog)  Indices=[1 0]  OutputSizes=1
  Selector1 : Selector  InputPortWidth=3  IndexOptions=Index vector (dialog)  Indices=3  OutputSizes=1
  Selector2 : Selector  InputPortWidth=3  IndexOptions=Index vector (dialog)  Indices=1  OutputSizes=1
  Selector3 : Selector  InputPortWidth=3  IndexOptions=Index vector (dialog)  Indices=2  OutputSizes=1
  Vector Concatenate : Concatenate  NumInputs=3
  FGInterface : Outport  VectorParamsAs1DForOutWhenUnconnected=off
  XYZ_NED : Outport  Port=2  VectorParamsAs1DForOutWhenUnconnected=off
  AttitudeQuaternion : Outport  Port=3  VectorParamsAs1DForOutWhenUnconnected=off
  wires:
  Mux1/1 -> FGInterface/1
  Constant/1 -> Flat Earth to LLA/2
  Bus Selector/1 -> Coordinate Transformation Conversion/1, Mux1/2  "<aircraftEulerAngles_rad>"
  Flat Earth to LLA/2 -> Mux/2
  Flat Earth to LLA/1 -> Selector/1
  Bus Selector1/1 -> [aircraftPosInNED_m], Flat Earth to LLA/1  "<aircraftPosInNED_m>"
  VehicleBus/1 -> Bus Selector/1, Bus Selector1/1
  Selector/1 -> Mux/1
  Mux/1 -> Selector1/1, Mux1/1
  Selector2/1 -> Vector Concatenate/1
  Selector3/1 -> Vector Concatenate/2
  Vector Concatenate/1 -> XYZ_NED/1
  Selector1/1 -> Gain/1
  Gain/1 -> Vector Concatenate/3
  [aircraftPosInNED_m] -> Selector3/1, Selector2/1
  Coordinate Transformation Conversion/1 -> AttitudeQuaternion/1  "Rotation"

== system VehicleSilSimulation/PX4 HITL Interface/HIL_GPS/GPS/GPS Time Update ==
  Timestamp : Inport
  Enable : EnablePort
  Update GPS Time : DataStoreWrite  DataStoreName=GPS  IndexOptions=Index vector (dialog)  Indices=1  OutputSizes=1
  wires:
  Timestamp/1 -> Update GPS Time/1

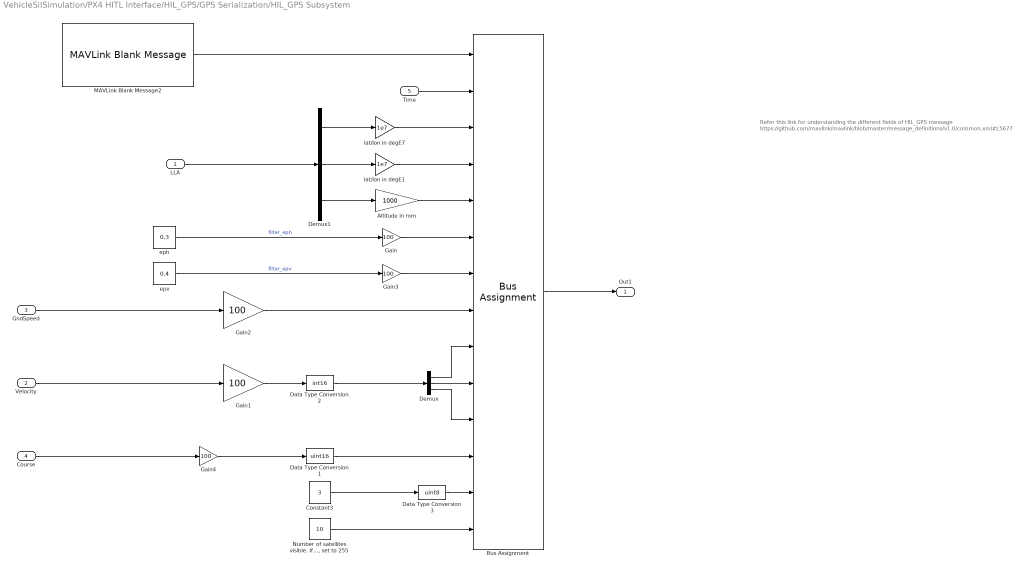
== system VehicleSilSimulation/PX4 HITL Interface/HIL_GPS/GPS Serialization/HIL_GPS Subsystem ==
  note: Refer this link for understanding the different fields of HIL_GPS message https://github.com/mavlink/mavlink/blob/master/message_definitions/v1.0/common.xml#L5677
  LLA : Inport
  Velocity : Inport  Port=2
  GndSpeed : Inport  Port=3
  Course : Inport  Port=4
  Time : Inport  Port=5
  Altitude in mm : Gain  Gain=1000  OutDataTypeStr=Inherit: Inherit via back propagation
  Bus Assignment : BusAssignment  AssignedSignals=Payload.time_usec,Payload.lat,Payload.lon,Payload.alt,Payload.eph,Payload.epv,Payload.vel,Payload.vn,Payload.ve,Payload.vd,Payload.cog,Payload.fix_type,Payload.satellites_visible
  Constant3 : Constant  Value=3  OutDataTypeStr=Inherit: Inherit via back propagation  SampleTime=-1
  Data Type Conversion1 : DataTypeConversion  OutDataTypeStr=uint16  SaturateOnIntegerOverflow=off  RndMeth=Floor
  Data Type Conversion2 : DataTypeConversion  OutDataTypeStr=int16  SaturateOnIntegerOverflow=off  RndMeth=Floor
  Data Type Conversion3 : DataTypeConversion  OutDataTypeStr=uint8  SaturateOnIntegerOverflow=off  RndMeth=Floor
  Demux : Demux  Outputs=3
  Demux1 : Demux  Outputs=3
  Gain : Gain  Gain=100  OutDataTypeStr=Inherit: Inherit via back propagation
  Gain1 : Gain  Gain=100
  Gain2 : Gain  Gain=100  OutDataTypeStr=uint16
  Gain3 : Gain  Gain=100  OutDataTypeStr=Inherit: Inherit via back propagation
  Gain4 : Gain  Gain=100
  MAVLink Blank Message2 : uavmavlinklib/MAVLink Blank Message  dialectSource=Select from standard MAVLink dialects  dialect=common.xml  dialectCustom=common.xml  version=2  messageType=HIL_GPS  SystemID=2  ComponentID=51  SampleTime=-1
  "Number of satellites visible. If unknown, set to 255" : Constant  Value=10  OutDataTypeStr=Inherit: Inherit via back propagation  SampleTime=-1
  eph : Constant  Value=0.3  SampleTime=-1
  epv : Constant  Value=0.4  SampleTime=-1
  lat/lon in degE1 : Gain  Gain=1e7  OutDataTypeStr=Inherit: Inherit via back propagation
  lat/lon in degE7 : Gain  Gain=1e7  OutDataTypeStr=Inherit: Inherit via back propagation
  Out1 : Outport
  wires:
  Gain2/1 -> Bus Assignment/8
  lat/lon in degE7/1 -> Bus Assignment/3
  Demux1/1 -> lat/lon in degE7/1
  Demux/3 -> Bus Assignment/11
  MAVLink Blank Message2/1 -> Bus Assignment/1
  Gain1/1 -> Data Type Conversion2/1
  Demux1/3 -> Altitude in mm/1
  Demux1/2 -> lat/lon in degE1/1
  Demux/1 -> Bus Assignment/9
  lat/lon in degE1/1 -> Bus Assignment/4
  Altitude in mm/1 -> Bus Assignment/5
  Data Type Conversion2/1 -> Demux/1
  Demux/2 -> Bus Assignment/10
  Gain/1 -> Bus Assignment/6
  Gain3/1 -> Bus Assignment/7
  GndSpeed/1 -> Gain2/1
  Velocity/1 -> Gain1/1
  Course/1 -> Gain4/1
  Data Type Conversion1/1 -> Bus Assignment/12
  eph/1 -> Gain/1  "filter_eph"
  epv/1 -> Gain3/1  "filter_epv"
  Data Type Conversion3/1 -> Bus Assignment/13
  Gain4/1 -> Data Type Conversion1/1
  Time/1 -> Bus Assignment/2
  LLA/1 -> Demux1/1
  Bus Assignment/1 -> Out1/1
  Constant3/1 -> Data Type Conversion3/1
  "Number of satellites visible. If unknown, set to 255"/1 -> Bus Assignment/14

== system VehicleSilSimulation/PX4 HITL Interface/Send Heartbeat/GPS/Heartbeat Time Update ==
  Timestamp : Inport
  Enable : EnablePort
  Update Heartbeat Time : DataStoreWrite  DataStoreName=Heartbeat  IndexOptions=Index vector (dialog)  Indices=1  OutputSizes=1
  wires:
  Timestamp/1 -> Update Heartbeat Time/1
